simulink model "ofdm"  (R2016a)
settings: Solver=VariableStepAuto  StartTime=0.0  StopTime=0.02  RelTol=1e-3
values from neighbouring files (symbols this model uses):
  A = 10    [Config.m]
  BW = F_SC*N    (= 50000000)    [Config.m]
  F_SC = 24414.0625*k    (= 195312.5)    [Config.m]
  K = 960    [Config.m]
  N = 256    [Config.m]
undefined symbols (not defined in the file or in its folder): R
libraries: commutil2 x2, commsequence2 x2, dspxfrm3 x1, commblkcod2 x1, dspsigops x1, commrflib2 x1, commdigbbndpm3 x1, commrandsrc3 x1
settings Model: Creator=Jsinno  LastModifiedBy=Jsinno

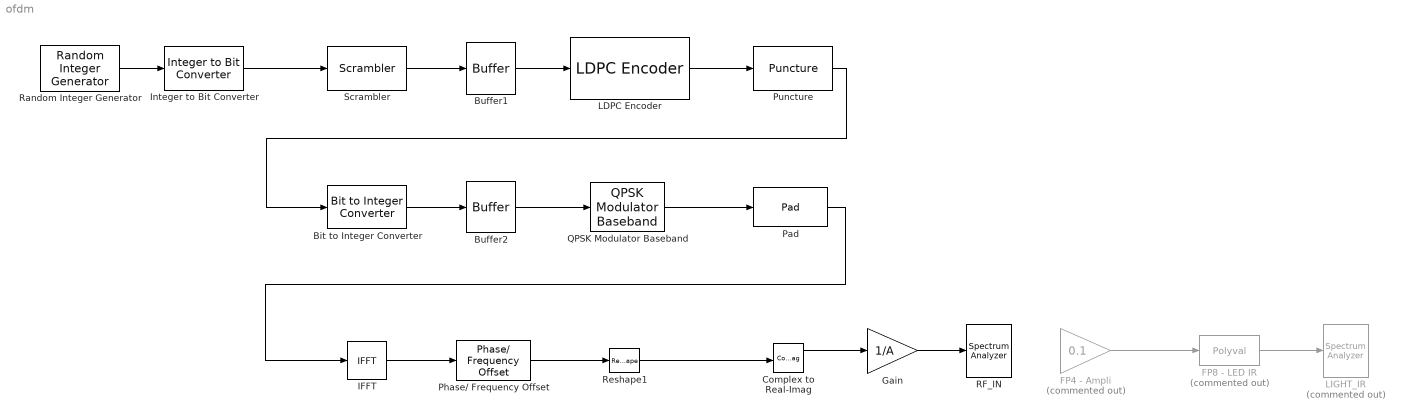
== system ofdm ==
  Bit to Integer Converter : commutil2/Bit to Integer Converter  nbits=2  bitOrder=MSB first  signedOutputValues=Unsigned  outDtype=Inherit via internal rule  outDtypeSigned=Inherit via internal rule
  Buffer1 : Buffer  N=K  TreatMby1Signals=One channel  OutputFrames=off
  Buffer2 : Buffer  N=256  TreatMby1Signals=One channel  OutputFrames=off
  Complex to Real-Imag : ComplexToRealImag
  FP4 - Ampli : Gain  Commented=on  Gain=0.1
  FP8 - LED IR : Polyval  Commented=on  Coefs=[-0.008931725655987,-0.026453643512349,0.983644029213939,0.904846032331364]
  Gain : Gain  Gain=1/A
  IFFT : dspxfrm3/IFFT  FFTImplementation=Auto  CompMethod=Table lookup  TableOpt=NEW  TableOptActive=Speed  BitRevOrder=off  cs_in=off  Normalize=off  InheritFFTLength=on  FFTLength=1024  WrapInput=off  mode=Complex  outSamplingMode=Sample based  roundingMode=Floor  overflowMode=off  firstCoeffDataTypeStr=Inherit: Same word length as input  firstCoeffLastDataTypeStr=Inherit: Same word length as input  outputMin=[]  outputMax=[]
  Integer to Bit Converter : commutil2/Integer to Bit Converter  nbits=2  signedInputValues=Unsigned  bitOrder=MSB first  outDtype=Inherit via internal rule
  LDPC Encoder : commblkcod2/LDPC Encoder  ParityCheckMat=H
  LIGHT_IR : SpectrumAnalyzer  Commented=on
  Pad : dspsigops/Pad  padAlong=Columns  dimsToPad=1  valSrc=Specify via dialog  padVal=0  spec=Output size  padNumOutRowsSpecMethod=User-specified  numOutRows=R*N  padNumOutColsSpecMethod=User-specified  numOutCols=256  isVarDimsMode=off  padBeginning=0  padEnd=0  outSizeMode=User-specified  outSize=1  padSigAt=Beginning and end  trunc_flag=None  roundingMode=Floor  overflowMode=off  truncOrWrapMode=Truncate  wrap_flag=None
  Phase/ Frequency Offset : commrflib2/Phase// Frequency Offset  phaseOffset=0  freqPort=off  freqOffset=R*BW
  Puncture : commsequence2/Puncture  punctureVector=[1 1 1 1 1 1 1 1 1 1 1 1 1 1 1 1] .'
  QPSK Modulator Baseband : commdigbbndpm3/QPSK Modulator Baseband  InType=Integer  Enc=Gray  Ph=pi/4  outDtype=double  outWordLen=16  outUDDataType=sfix(16)  outFracLenMode=Best precision  outFracLen=15  outDataTypeStr=double  outLastDataTypeStr=double
  RF_IN : SpectrumAnalyzer
  Random Integer Generator : commrandsrc3/Random Integer Generator  SetSize=4  SeedSource=Auto  Seed=0  SampleTime=1/(N*F_SC)  SamplesPerFrame=K/2  OutputDataType=uint8  SimulateUsing=Interpreted execution
  Reshape1 : Reshape  OutputDimensions=[512,1]
  Scrambler : commsequence2/Scrambler  M=2  poly='1 + z^-18 + z^-23'  iniStaSource=Dialog Parameter  ini_sta=[1 0 1 0 1 0 1 0 1 0 1 0 1 0 1 0 1 0 1 0 1 0 1]  resetViaPort=off
  wires:
  Pad/1 -> IFFT/1
  IFFT/1 -> Phase/ Frequency Offset/1
  Phase/ Frequency Offset/1 -> Reshape1/1
  FP8 - LED IR/1 -> LIGHT_IR/1
  FP4 - Ampli/1 -> FP8 - LED IR/1
  Gain/1 -> RF_IN/1
  QPSK Modulator Baseband/1 -> Pad/1
  Reshape1/1 -> Complex to Real-Imag/1
  Complex to Real-Imag/1 -> Gain/1
  Random Integer Generator/1 -> Integer to Bit Converter/1
  Integer to Bit Converter/1 -> Scrambler/1
  LDPC Encoder/1 -> Puncture/1
  Scrambler/1 -> Buffer1/1
  Buffer1/1 -> LDPC Encoder/1
  Bit to Integer Converter/1 -> Buffer2/1
  Buffer2/1 -> QPSK Modulator Baseband/1
  Puncture/1 -> Bit to Integer Converter/1
